simulink model "Kurs"  (R2024a)
settings: Solver=ode1  StartTime=0.0  StopTime=1.2  FixedStep=0.000001  RelTol=1e-3
InitFcn:
  | Kpr = 56;
  | Tpr = 0.002;
  | Rya = 1.78;
  | Tya = 0.16;
  | c = 0.56;
  | J = 0.05;
  | Kot = 0.054;
  | Koc = 0.09;
  | T1 = 0.0013;
  | T2 = 0.0165;
  | T4 = 0.207;
  | K1 = 6.74;
  | K2 = 3.12;
  | K3 = 0.874;
  | X1max = 3;
  | Y2max = 250;
  | Y4max = 90;
  | Z = 17;
  | treg = 0.001;
  | toy = 0.0001;
undefined symbols (not defined in the file or in its folder): Kaw, tre
libraries: slpidlib x5
(part 1 of 2)
settings Model: Creator=nicki  LastModifiedBy=nicki
settings RTWCC: GPUComputeCapability=3.5

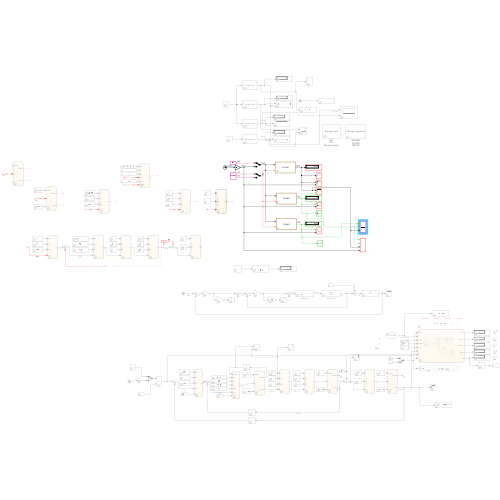
[thumbnail: Simulink's stored preview of the top-level diagram]
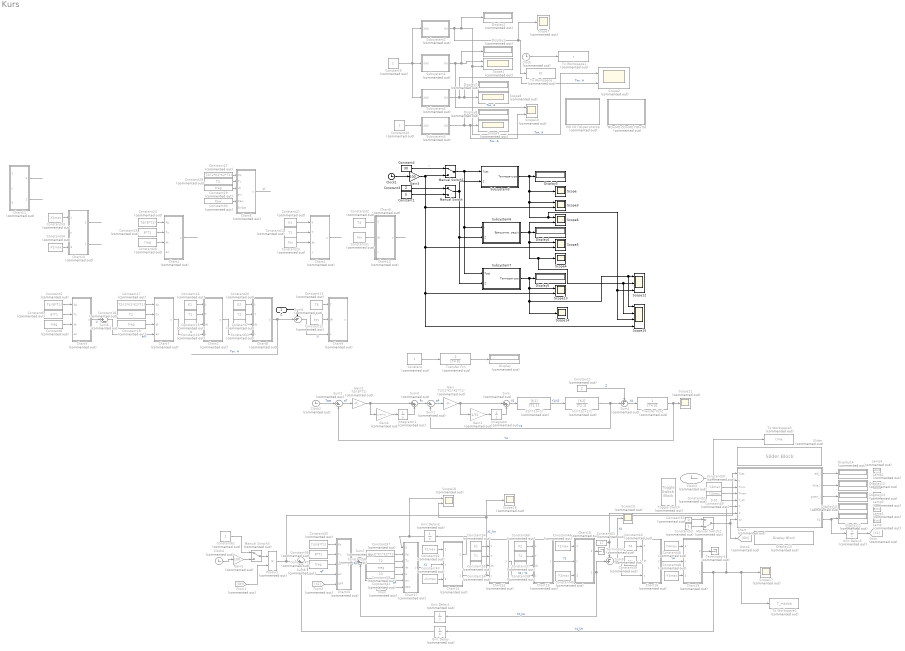
== system Kurs ==
  Z : Inport
  Chart : Stateflow chart  Commented=on  TreatAsAtomicUnit=on  SystemSampleTime=treg
      settings: PortSchema="{\"entries\":[{\"content\":{\"sides\":[{\"content\":{\"connectorIds\":[\"In8\",\"In1\",\"In2\",\"In3\",\"In5\",\"In4\",\"In6\",\"In7\"]},\"type\":\"ConnectorPlacement.EquallySpacedRectSide\",\"uuid\":\"2a18dcd6-4b0c-4a76-a20c-2dc316dd2b01\"},{\"content\":{\"connectorIds\":[\"Out1\",\"Out2\",\"Out3\",\"Out4\",\"Out5\"],\"side\":\"RIGHT\"},\"type\":\"ConnectorPlacement.EquallySpacedRectSide\",\"uuid\":\"9e7f62ff-8b1d-44fe-8b34-5f319205903d\"},{\"content\":{\"side\":\"TOP\"},\"type\":\"ConnectorPlacement.EquallySpacedRectSide\",\"uuid\":\"488e4df1-10a7-4056-869a-c48ac259fb0e\"}]},\"type\":\"ConnectorPlacement.EquallySpacedConnector\",\"uuid\":\"21634ba7-0beb-4d40-a7b7-ac3b35c407ea\"}],\"packageUris\":[\"http://schema.mathworks.com/mf0/Connector/R2020b\"],\"version\":\"1.0\"}"
  Chart1 : Stateflow chart  Commented=on  TreatAsAtomicUnit=on  SystemSampleTime=treg
  Chart10 : Stateflow chart  Commented=on  TreatAsAtomicUnit=on  SystemSampleTime=treg
      settings: PortSchema="{\"entries\":[{\"content\":{\"sides\":[{\"content\":{\"connectorIds\":[\"In1\",\"In2\",\"In3\"]},\"type\":\"ConnectorPlacement.EquallySpacedRectSide\",\"uuid\":\"06dc2d10-fdc8-420b-b9cd-f5fc9c52f6ec\"},{\"content\":{\"connectorIds\":[\"Out2\",\"Out1\"],\"side\":\"RIGHT\"},\"type\":\"ConnectorPlacement.EquallySpacedRectSide\",\"uuid\":\"6c618a25-ba21-4ff8-999c-a9529d925b85\"},{\"content\":{\"side\":\"TOP\"},\"type\":\"ConnectorPlacement.EquallySpacedRectSide\",\"uuid\":\"fb5392fe-c913-4872-919e-93e45aee3608\"}]},\"type\":\"ConnectorPlacement.EquallySpacedConnector\",\"uuid\":\"af73c6a6-6f26-4653-9043-b34907f5f2e4\"}],\"packageUris\":[\"http://schema.mathworks.com/mf0/Connector/R2020b\"],\"version\":\"1.0\"}"
  Chart11 : Stateflow chart  Commented=on  TreatAsAtomicUnit=on  SystemSampleTime=treg
      settings: PortSchema="{\"entries\":[{\"content\":{\"sides\":[{\"content\":{\"connectorIds\":[\"In1\",\"In2\",\"In3\"]},\"type\":\"ConnectorPlacement.EquallySpacedRectSide\",\"uuid\":\"06dc2d10-fdc8-420b-b9cd-f5fc9c52f6ec\"},{\"content\":{\"connectorIds\":[\"Out2\",\"Out1\"],\"side\":\"RIGHT\"},\"type\":\"ConnectorPlacement.EquallySpacedRectSide\",\"uuid\":\"6c618a25-ba21-4ff8-999c-a9529d925b85\"},{\"content\":{\"side\":\"TOP\"},\"type\":\"ConnectorPlacement.EquallySpacedRectSide\",\"uuid\":\"fb5392fe-c913-4872-919e-93e45aee3608\"}]},\"type\":\"ConnectorPlacement.EquallySpacedConnector\",\"uuid\":\"af73c6a6-6f26-4653-9043-b34907f5f2e4\"}],\"packageUris\":[\"http://schema.mathworks.com/mf0/Connector/R2020b\"],\"version\":\"1.0\"}"
  Chart12 : Stateflow chart  Commented=on  TreatAsAtomicUnit=on  SystemSampleTime=toy
  Chart13 : Stateflow chart  Commented=on  TreatAsAtomicUnit=on  SystemSampleTime=toy
  Chart14 : Stateflow chart  Commented=on  TreatAsAtomicUnit=on  SystemSampleTime=treg
      settings: PortSchema="{\"entries\":[{\"content\":{\"sides\":[{\"content\":{\"connectorIds\":[\"In1\",\"In2\",\"In3\"]},\"type\":\"ConnectorPlacement.EquallySpacedRectSide\",\"uuid\":\"06dc2d10-fdc8-420b-b9cd-f5fc9c52f6ec\"},{\"content\":{\"connectorIds\":[\"Out2\",\"Out1\"],\"side\":\"RIGHT\"},\"type\":\"ConnectorPlacement.EquallySpacedRectSide\",\"uuid\":\"6c618a25-ba21-4ff8-999c-a9529d925b85\"},{\"content\":{\"side\":\"TOP\"},\"type\":\"ConnectorPlacement.EquallySpacedRectSide\",\"uuid\":\"fb5392fe-c913-4872-919e-93e45aee3608\"}]},\"type\":\"ConnectorPlacement.EquallySpacedConnector\",\"uuid\":\"af73c6a6-6f26-4653-9043-b34907f5f2e4\"}],\"packageUris\":[\"http://schema.mathworks.com/mf0/Connector/R2020b\"],\"version\":\"1.0\"}"
  Chart15 : Stateflow chart  Commented=on  TreatAsAtomicUnit=on  SystemSampleTime=toy
  Chart16 : Stateflow chart  Commented=on  TreatAsAtomicUnit=on  SystemSampleTime=toy
  Chart17 : Stateflow chart  Commented=on  TreatAsAtomicUnit=on  SystemSampleTime=treg
      settings: PortSchema="{\"entries\":[{\"content\":{\"sides\":[{\"content\":{\"connectorIds\":[\"In5\",\"In1\",\"In2\",\"In3\",\"In6\",\"In4\",\"In7\"]},\"type\":\"ConnectorPlacement.EquallySpacedRectSide\",\"uuid\":\"b164ad06-1259-4e4e-9be1-6467b125c0e4\"},{\"content\":{\"connectorIds\":[\"Out1\"],\"side\":\"RIGHT\"},\"type\":\"ConnectorPlacement.EquallySpacedRectSide\",\"uuid\":\"0593e984-4c4d-48f3-925e-b61cefc7aa48\"},{\"content\":{\"side\":\"TOP\"},\"type\":\"ConnectorPlacement.EquallySpacedRectSide\",\"uuid\":\"e7a407e5-6ce2-46ef-876b-9c67a31d7a68\"}]},\"type\":\"ConnectorPlacement.EquallySpacedConnector\",\"uuid\":\"345a9212-fd2f-406e-95cd-4fdf60a3ef4b\"}],\"packageUris\":[\"http://schema.mathworks.com/mf0/Connector/R2020b\"],\"version\":\"1.0\"}"
  Chart18 : Stateflow chart  Commented=on  TreatAsAtomicUnit=on  SystemSampleTime=toy
      settings: PortSchema="{\"entries\":[{\"content\":{\"sides\":[{\"content\":{\"connectorIds\":[\"In1\",\"In2\",\"In3\"]},\"type\":\"ConnectorPlacement.EquallySpacedRectSide\",\"uuid\":\"06dc2d10-fdc8-420b-b9cd-f5fc9c52f6ec\"},{\"content\":{\"connectorIds\":[\"Out2\",\"Out1\"],\"side\":\"RIGHT\"},\"type\":\"ConnectorPlacement.EquallySpacedRectSide\",\"uuid\":\"6c618a25-ba21-4ff8-999c-a9529d925b85\"},{\"content\":{\"side\":\"TOP\"},\"type\":\"ConnectorPlacement.EquallySpacedRectSide\",\"uuid\":\"fb5392fe-c913-4872-919e-93e45aee3608\"}]},\"type\":\"ConnectorPlacement.EquallySpacedConnector\",\"uuid\":\"af73c6a6-6f26-4653-9043-b34907f5f2e4\"}],\"packageUris\":[\"http://schema.mathworks.com/mf0/Connector/R2020b\"],\"version\":\"1.0\"}"
  Chart19 : Stateflow chart  Commented=on  TreatAsAtomicUnit=on  SystemSampleTime=toy
      settings: PortSchema="{\"entries\":[{\"content\":{\"sides\":[{\"content\":{\"connectorIds\":[\"In1\",\"In2\",\"In3\"]},\"type\":\"ConnectorPlacement.EquallySpacedRectSide\",\"uuid\":\"06dc2d10-fdc8-420b-b9cd-f5fc9c52f6ec\"},{\"content\":{\"connectorIds\":[\"Out2\",\"Out1\"],\"side\":\"RIGHT\"},\"type\":\"ConnectorPlacement.EquallySpacedRectSide\",\"uuid\":\"6c618a25-ba21-4ff8-999c-a9529d925b85\"},{\"content\":{\"side\":\"TOP\"},\"type\":\"ConnectorPlacement.EquallySpacedRectSide\",\"uuid\":\"fb5392fe-c913-4872-919e-93e45aee3608\"}]},\"type\":\"ConnectorPlacement.EquallySpacedConnector\",\"uuid\":\"af73c6a6-6f26-4653-9043-b34907f5f2e4\"}],\"packageUris\":[\"http://schema.mathworks.com/mf0/Connector/R2020b\"],\"version\":\"1.0\"}"
  Chart2 : Stateflow chart  Commented=on  TreatAsAtomicUnit=on  SystemSampleTime=toy
  Chart20 : Stateflow chart  Commented=on  TreatAsAtomicUnit=on  SystemSampleTime=treg
  Chart3 : Stateflow chart  Commented=on  TreatAsAtomicUnit=on  SystemSampleTime=treg
  Chart4 : Stateflow chart  Commented=on  TreatAsAtomicUnit=on  SystemSampleTime=toy
  Chart5 : Stateflow chart  Commented=on  TreatAsAtomicUnit=on  SystemSampleTime=toy
  Chart6 : Stateflow chart  Commented=on  TreatAsAtomicUnit=on  SystemSampleTime=treg
      settings: PortSchema="{\"entries\":[{\"content\":{\"sides\":[{\"content\":{\"connectorIds\":[\"In1\",\"In2\",\"In3\",\"In4\",\"In6\",\"In5\"]},\"type\":\"ConnectorPlacement.EquallySpacedRectSide\",\"uuid\":\"b164ad06-1259-4e4e-9be1-6467b125c0e4\"},{\"content\":{\"connectorIds\":[\"Out1\"],\"side\":\"RIGHT\"},\"type\":\"ConnectorPlacement.EquallySpacedRectSide\",\"uuid\":\"0593e984-4c4d-48f3-925e-b61cefc7aa48\"},{\"content\":{\"side\":\"TOP\"},\"type\":\"ConnectorPlacement.EquallySpacedRectSide\",\"uuid\":\"e7a407e5-6ce2-46ef-876b-9c67a31d7a68\"}]},\"type\":\"ConnectorPlacement.EquallySpacedConnector\",\"uuid\":\"345a9212-fd2f-406e-95cd-4fdf60a3ef4b\"}],\"packageUris\":[\"http://schema.mathworks.com/mf0/Connector/R2020b\"],\"version\":\"1.0\"}"
  Chart7 : Stateflow chart  Commented=on  TreatAsAtomicUnit=on  SystemSampleTime=treg
  Chart8 : Stateflow chart  Commented=on  TreatAsAtomicUnit=on  SystemSampleTime=toy
  Chart9 : Stateflow chart  Commented=on  TreatAsAtomicUnit=on  SystemSampleTime=toy
  Clock{,2..4} (4 alike) : Clock  Commented=on
  Clock1 : Clock
  Constant{,9..10,52,61} (5 alike) : Constant  Commented=on
  Constant1 : Constant  Value=0
  Constant{11..12,16,23,31,38..39,56} (8 alike) : Constant  Commented=on  Value=toy
  Constant13 : Constant  Commented=on  Value=T4
  Constant14 : Constant  Commented=on  Value=K1
  Constant15 : Constant  Commented=on  Value=T1
  Constant17 : Constant  Commented=on  Value=T2/(2*K1*K2*T1)
  Constant{7,18,28,37,58} (5 alike) : Constant  Commented=on  Value=T2
  Constant{8,19,26,29,47,59} (6 alike) : Constant  Commented=on  Value=treg
  Constant2 : Constant  Commented=on  Value=Z
  Constant20 : Constant  Commented=on  Value=K2
  Constant21 : Constant  Commented=on  Value=K1
  Constant22 : Constant  Commented=on  Value=T1
  Constant24 : Constant  Commented=on  Value=T4/(8*T1)
  Constant25 : Constant  Commented=on  Value=8*T1
  Constant27 : Constant  Commented=on  Value=T2/(2*K1*K2*T1)
  Constant3 : Constant  Value=Z
  Constant30 : Constant  Commented=on  Value=Kaw
  Constant32 : Constant  Commented=on  Value=T4
  Constant33 : Constant  Commented=on  Value=X1max
  Constant34 : Constant  Commented=on  Value=-X1max
  Constant35 : Constant  Commented=on  Value=T4/(8*T1)
  Constant36 : Constant  Commented=on  Value=8*T1
  Constant4 : Constant  Value=30
  Constant40 : Constant  Commented=on  Value=T4
  Constant41 : Constant  Commented=on  Value=10
  Constant42 : Constant  Commented=on  Value=X1max
  Constant43 : Constant  Commented=on  Value=-X1max
  Constant44 : Constant  Commented=on  Value=Y2max
  Constant45 : Constant  Commented=on  Value=-Y2max
  Constant46 : Constant  Commented=on  Value=Y4max
  Constant48 : Constant  Commented=on  Value=-Y4max
  Constant49 : Constant  Commented=on  Value=Y4max
  Constant5 : Constant  Commented=on  Value=T4/(8*T1)
  Constant50 : Constant  Commented=on  Value=-Y4max
  Constant51 : Constant  Commented=on  Value=0.01
  Constant53 : Constant  Commented=on  Value=0
  Constant54 : Constant  Commented=on  Value=K1
  Constant55 : Constant  Commented=on  Value=T1
  Constant57 : Constant  Commented=on  Value=T2/(2*K1*K2*T1)
  Constant6 : Constant  Commented=on  Value=8*T1
  Constant60 : Constant  Commented=on  Value=K2
  Constant62 : Constant  Commented=on  Value=17
  Display{,1..2,7..8,10..14} (10 alike) : Display  Commented=on
  Display15 : DisplayBlock  Commented=on  LabelPosition=Hide  Transparency=1
  Display3 : Display
  Display4 : Display
  Display5 : Display
  From : From  Commented=on  GotoTag=X1
  From1 : From  Commented=on  GotoTag=ON
  From2 : From  Commented=on  GotoTag=X1
  Gain : Gain  Commented=on  Gain=T2/(2*K1*K2*T1)
  Gain1 : Gain  Commented=on  Gain=1/T2
  Gain2 : Gain  Commented=on  Gain=T4/(8*T1)
  Gain3 : Gain  Gain=100
  Gain4 : Gain  Commented=on  Gain=1/(8*T1)
  Gain5 : Gain  Commented=on  Gain=100
  Goto : Goto  Commented=on  GotoTag=X1
  Goto1 : Goto  Commented=on  GotoTag=ON
  Integrator : Integrator  Commented=on
  Integrator1 : Integrator  Commented=on
  Lamp : LampBlock  Commented=on  LabelPosition=Hide  Icon=Check1
  Lamp1 : LampBlock  Commented=on  LabelPosition=Hide  Icon=Check1
  Lamp2 : LampBlock  Commented=on  LabelPosition=Hide
  Lamp3 : LampBlock  Commented=on  LabelPosition=Hide
  Lamp4 : LampBlock  Commented=on  LabelPosition=Hide
  Manual Switch : ManualSwitch
  Manual Switch1 : ManualSwitch
  Manual Switch2 : ManualSwitch  Commented=on  CurrentSetting=0
  Manual Switch3 : ManualSwitch  Commented=on
  Product : Product  Commented=on
  Scope : Scope
  Scope{1..2,10,18} (4 alike) : Scope  Commented=on  NumInputPorts=2
  Scope{7..9,11,16..17,19} (7 alike) : Scope  Commented=on
  Scope12 : Scope  NumInputPorts=3
  Scope{3,5..6,13} (4 alike) : Scope  NumInputPorts=2
  Scope14 : Scope
  Scope15 : Scope  NumInputPorts=4
  Scope4 : Scope
  Slider : SliderBlock  Commented=on  ScaleMin=-100
  Subsystem1 : Subsystem  Commented=on  mask{Kpr=Kpr, Tpr=Tpr, Rya=Rya, Tya=Tya, Cm=c, Ce=c, Kot=Kot, Koc=Koc, treg=1/1000, toy=1 / 10000}
      mask prompts: Kpr "Коэффициент усиления преобразователя"; Tpr "Постоянная времени преобразователя"; Rya "Коэффициент усиления тока (1/Rya)"; Tya "Постоянная времени тока"; Cm "Постоянный конструктивный коэффициент (коэффициент связи)"; Ce "Постоянный конструктивный коэффициент (u = Ce*w)"; Kot "Коэффициент обратной связи тока"; Koc "Коэффициент обратной связи угловой скорости"; treg "Шаг дискретизации регуляторов"; toy "Шаг дискретизации ОУ"
      mask Display: disp('Контур тока');
  Subsystem2 : Subsystem  Commented=on  mask{Kpr=Kpr, Tpr=Tpr, Rya=Rya, Tya=Tya, Cm=c, Ce=c, Kot=Kot, Koc=Koc, treg=1/1000, toy=1 / 10000}
      mask prompts: Kpr "Коэффициент усиления преобразователя"; Tpr "Постоянная времени преобразователя"; Rya "Коэффициент усиления тока (1/Rya)"; Tya "Постоянная времени тока"; Cm "Постоянный конструктивный коэффициент (коэффициент связи)"; Ce "Постоянный конструктивный коэффициент (u = Ce*w)"; Kot "Коэффициент обратной связи тока"; Koc "Коэффициент обратной связи угловой скорости"; treg "Шаг дискретизации регуляторов"; toy "Шаг дискретизации ОУ"
      mask Display: disp('Контур тока');
  Subsystem3 : Subsystem
      mask Display: disp('СО+МО');
  Subsystem4 : Subsystem  Commented=on  mask{Kpr=Kpr, Tpr=Tpr, Rya=Rya, Tya=Tya, Cm=c, Ce=c, Kot=Kot, Koc=Koc, treg=1/1000, toy=1 / 10000}
      mask prompts: Kpr "Коэффициент усиления преобразователя"; Tpr "Постоянная времени преобразователя"; Rya "Коэффициент усиления тока (1/Rya)"; Tya "Постоянная времени тока"; Cm "Постоянный конструктивный коэффициент (коэффициент связи)"; Ce "Постоянный конструктивный коэффициент (u = Ce*w)"; Kot "Коэффициент обратной связи тока"; Koc "Коэффициент обратной связи угловой скорости"; treg "Шаг дискретизации регуляторов"; toy "Шаг дискретизации ОУ"
      mask Display: disp('Контур тока');
  Subsystem5 : Subsystem  Commented=on  mask{Kpr=Kpr, Tpr=Tpr, Rya=Rya, Tya=Tya, Cm=c, Ce=c, Kot=Kot, Koc=Koc, treg=1/1000, toy=1 / 10000}
      mask prompts: Kpr "Коэффициент усиления преобразователя"; Tpr "Постоянная времени преобразователя"; Rya "Коэффициент усиления тока (1/Rya)"; Tya "Постоянная времени тока"; Cm "Постоянный конструктивный коэффициент (коэффициент связи)"; Ce "Постоянный конструктивный коэффициент (u = Ce*w)"; Kot "Коэффициент обратной связи тока"; Koc "Коэффициент обратной связи угловой скорости"; treg "Шаг дискретизации регуляторов"; toy "Шаг дискретизации ОУ"
      mask Display: disp('ПИ (дискрет)');
  Subsystem6 : Subsystem
      mask Display: disp('СО+МО');
  Subsystem7 : Subsystem
      mask Display: disp('СО+МО');
  Sum : Sum  Commented=on  Inputs=|++
  Sum{1..2,5,7..8} (5 alike) : Sum  Commented=on  Inputs=|+-
  Sum3 : Sum  Commented=on  Inputs=|++
  Sum4 : Sum  Commented=on  Inputs=-+|
  Sum6 : Sum  Commented=on  Inputs=-+|
  Sum9 : Sum  Commented=on  Inputs=-+|
  Terminator : Terminator  Commented=on
  Terminator1 : Terminator  Commented=on
  To Workspace : ToWorkspace  Commented=on  VariableName=Kt  SampleTime=0.001
  To Workspace1 : ToWorkspace  Commented=on  VariableName=t  SampleTime=0.001
  To Workspace2 : ToWorkspace  Commented=on  VariableName=T_matlab  SampleTime=0.002
  To Workspace3 : ToWorkspace  Commented=on  VariableName=time  SampleTime=0.002
  Toggle Switch : ToggleSwitchBlock  Commented=on
      settings: Values={{'Off', 'On'}, [17 0]}
  Transfer Fcn : TransferFcn  Commented=on  Denominator=[T4 0]
  Transfer Fcn1 : TransferFcn  Commented=on  Denominator=[T4 0]
  Unit Delay{,1..3} (4 alike) : UnitDelay  Commented=on  SampleTime=treg  HasFrameUpgradeWarning=on
  k1/(T1s+1) : TransferFcn  Commented=on  Numerator=[K1]  Denominator=[T1 1]
  k1/(T1s+1)1 : TransferFcn  Commented=on  Numerator=[K2]  Denominator=[T2 1]
  МО СО ПИ-регулятор : Subsystem  Commented=on
      mask Display: disp('Контур тока');
  МО+МО СО+МО ПИ+ПИ : Subsystem  Commented=on
      mask Display: disp('Контур скорости');
  wires:
  Subsystem4/1(I(t)) -> Scope2/2, Display7/1, Scope8/1  "Ток, А"
  Subsystem5/1(I(t)) -> Display8/1, Scope10/2, Scope9/1  "Ток, А"
  Constant10/1 -> Subsystem5/1(i0(t))
  Subsystem1/1(I(t)) -> Scope10/1, Display1/1, Scope1/1  "Ток, А"
  Constant9/1 -> Subsystem4/1(i0(t)), Subsystem2/1(i0(t)), Subsystem1/1(i0(t))
  Subsystem2/1(I(t)) -> Scope7/1, To Workspace/1, Display2/1, Scope1/2, Scope2/1  "Ток, А"
  Clock/1 -> To Workspace1/1
  Manual Switch1/1 -> Subsystem7/1(Tset), Subsystem6/1(i), Subsystem3/1(Tset)
  Manual Switch/1 -> Subsystem7/2(Z), Subsystem6/2(Z), Subsystem3/2(Z)
  Constant1/1 -> Manual Switch/2
  Constant3/1 -> Manual Switch/1
  Subsystem3/1(Температура) -> Display3/1, Scope15/3, Scope12/3, Scope6/1, Scope3/1, Scope/1
  Constant4/1 -> Manual Switch1/1  "i"
  Subsystem6/1("Вращение, рад/с") -> Scope6/2, Scope15/2, Scope12/2, Scope4/1, Scope5/1, Display4/1
  Constant/1 -> Transfer Fcn/1
  Transfer Fcn/1 -> Display/1
  Integrator1/1 -> Sum3/2
  Gain2/1 -> Sum3/1, Gain4/1
  Gain4/1 -> Integrator1/1
  k1/(T1s+1)/1 -> k1/(T1s+1)1/1  "Y1/X2"
  Gain/1 -> Gain1/1, Sum/1
  Constant2/1 -> Sum4/1  "Z"
  Sum4/1 -> Transfer Fcn1/1  "X4"
  Transfer Fcn1/1 -> Scope11/1, Sum2/2  "Y4"
  Sum1/1 -> Gain/1  "eP"
  Clock2/1 -> Sum2/1  "Tset"
  Sum2/1 -> Gain2/1  "eT"
  Gain1/1 -> Integrator/1
  Sum/1 -> k1/(T1s+1)/1  "X1"
  k1/(T1s+1)1/1 -> Sum4/2, Sum1/2  "Y2"
  Integrator/1 -> Sum/2
  Sum3/1 -> Sum1/1  "Pn"
  Subsystem7/1(Температура) -> Scope14/1, Scope15/1, Scope12/1, Scope13/1, Display5/1
  Clock1/1 -> Gain3/1
  Chart7/1(y) -> Chart2/4(x)  "U"
  Chart2/1(y) -> Chart8/4(x)
  ? -> Sum5/2
  Chart8/1(y) -> Sum6/2  "Ток, А"
  ? -> Chart3/4(err)  "e(i)"
  Constant18/1 -> Chart7/2(Tu)
  Constant12/1 -> Chart9/2(dt)
  Constant11/1 -> Chart8/3(dt)
  Constant20/1 -> Chart8/1(k)
  Constant13/1 -> Chart9/1(T)
  Constant19/1 -> Chart7/3(dt)
  Constant15/1 -> Chart2/2(T)
  Constant16/1 -> Chart2/3(dt)
  Z/1 -> Sum6/1
  Constant7/1 -> Chart8/2(T)
  Constant8/1 -> Chart3/3(dt)
  Constant5/1 -> Chart3/1(Kp)
  Sum6/1 -> Chart9/3(x)  "U"
  Constant17/1 -> Chart7/1(Kp)
  Chart3/1(y) -> Sum5/1  "U"
  Sum5/1 -> Chart7/4(err)  "e(i)"
  Constant6/1 -> Chart3/2(Tu)
  Constant14/1 -> Chart2/1(k)
  Constant21/1 -> Chart4/1(k)
  Constant22/1 -> Chart4/2(T)
  Constant23/1 -> Chart4/3(dt)
  ? -> Chart4/4(x)
  Chart4/1(y) -> ?
  Constant24/1 -> Chart1/1(Kp)
  Constant25/1 -> Chart1/2(Tu)
  Constant26/1 -> Chart1/3(dt)
  ? -> Chart1/4(err)
  Chart1/1(y) -> ?
  Constant27/1 -> Chart6/1(Kp)
  Constant28/1 -> Chart6/2(Tu)
  Constant29/1 -> Chart6/3(dt)
  Constant30/1 -> Chart6/6(Kaw)
  ? -> Chart6/4(err)
  ? -> Chart6/5(ErrSat)
  Chart6/1(y) -> ?  "U"
  Constant32/1 -> Chart5/1(T)
  Constant31/1 -> Chart5/2(dt)
  Chart5/1(y) -> ?
  ? -> Chart5/3(x)
  Constant34/1 -> Chart10/3(Ymin)
  Constant33/1 -> Chart10/1(Ymax)
  ? -> Chart10/2(y)  "U"
  Chart10/2(ErrSat) -> ?
  Chart10/1(y_lim) -> ?
  Chart11/1(y_lim) -> ?
  ? -> Chart11/2(y)  "U"
  Chart11/2(ErrSat) -> ?
  Gain3/1 -> Manual Switch1/2, Scope3/2, Scope15/4, Scope13/2, Scope5/2
  Constant50/1 -> Chart/2(Tmin)
  Product/1 -> Chart/8(Tset), Sum8/1
  Constant52/1 -> Manual Switch2/2
  From2/1 -> Chart20/5(OFF)
  From1/1 -> Product/2
  Chart/1(red_l) -> Display14/1
  Clock3/1 -> To Workspace3/1, Chart/1(t)
  Constant51/1 -> Chart/5(T_dz)
  Unit Delay3/1 -> Goto/1
  Chart14/2(ErrSat) -> Unit Delay2/1
  Constant48/1 -> Chart19/3(Ymin)
  Constant49/1 -> Chart/3(Tmax)
  Constant53/1 -> Manual Switch2/1
  Chart19/2(ErrSat) -> Terminator1/1
  Chart/3(green_l) -> Display13/1
  Unit Delay1/1 -> Sum7/2
  Chart18/2(ErrSat) -> Terminator/1
  Clock4/1 -> Gain5/1
  Constant37/1 -> Chart15/2(T)
  Constant44/1 -> Chart18/1(Ymax)
  Constant43/1 -> Chart14/3(Ymin)
  From/1 -> Chart17/7(OFF)
  Sum8/1 -> Chart20/4(err)  "eT"
  Constant54/1 -> Chart12/1(k)
  Constant46/1 -> Chart19/1(Ymax)
  Chart19/1(y_lim) -> To Workspace2/1, Scope17/1, Chart/4(T), Unit Delay/1  "Y4_lim"
  Chart16/1(y) -> Chart19/2(y)  "Y4"
  Constant55/1 -> Chart12/2(T)
  Manual Switch2/1 -> Goto1/1, Chart/7(on)
  Constant60/1 -> Chart15/1(k)
  Chart15/1(y) -> Chart18/2(y)  "Y2"
  Constant57/1 -> Chart17/1(Kp)
  Constant56/1 -> Chart12/3(dt)
  Constant40/1 -> Chart16/1(T)
  Unit Delay2/1 -> Scope18/1, Chart17/5(ErrSat)
  Constant59/1 -> Chart17/3(dt)
  Constant58/1 -> Chart17/2(Tu)
  Chart/4(error) -> Display10/1
  Constant42/1 -> Chart14/1(Ymax)
  Chart/5(X1) -> Display11/1, Unit Delay3/1
  Unit Delay/1 -> Sum8/2
  Constant45/1 -> Chart18/3(Ymin)
  Chart14/1(y_lim) -> Scope18/2, Scope16/1, Chart12/4(x)  "X1_lim"
  Chart18/1(y_lim) -> Unit Delay1/1, Sum9/2  "Y2_lim"
  Constant39/1 -> Chart16/2(dt)
  Chart17/1(y) -> Chart14/2(y)  "X1"
  Constant38/1 -> Chart15/3(dt)
  Constant47/1 -> Chart20/3(dt)
  Constant62/1 -> Sum9/1, Chart/6(Z)
  Chart12/1(y) -> Chart15/4(x)  "X2 / Y1"
  Constant36/1 -> Chart20/2(Tu)
  Constant35/1 -> Chart20/1(Kp)
  Chart20/1(y) -> Sum7/1  "Pn"
  Constant41/1 -> Chart17/6(Kaw)
  Sum9/1 -> Scope19/1, Chart16/3(x)  "X4"
  Sum7/1 -> Chart17/4(err)  "eP"
  Chart/2(blue_l) -> Display12/1
  Manual Switch3/1 -> Product/1
  Gain5/1 -> Manual Switch3/2
  Constant61/1 -> Manual Switch3/1

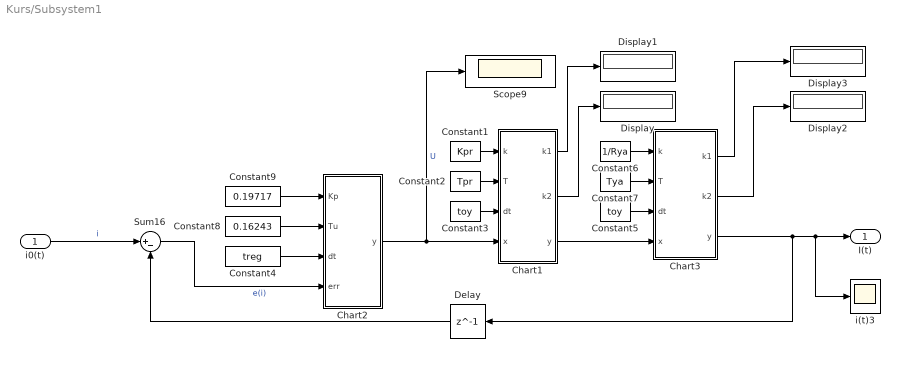
== system Kurs/Subsystem1 ==
  i0(t) : Inport
  Chart1 : Stateflow chart  TreatAsAtomicUnit=on  SystemSampleTime=toy
      settings: PortSchema="{\"entries\":[{\"content\":{\"sides\":[{\"content\":{\"connectorIds\":[\"In1\",\"In2\",\"In3\",\"In4\"]},\"type\":\"ConnectorPlacement.EquallySpacedRectSide\",\"uuid\":\"36dbee36-691d-4a1c-ac9a-2338e443d86d\"},{\"content\":{\"connectorIds\":[\"Out2\",\"Out3\",\"Out1\"],\"side\":\"RIGHT\"},\"type\":\"ConnectorPlacement.EquallySpacedRectSide\",\"uuid\":\"ede5d785-9ed8-4f22-af08-79b1e7897644\"},{\"content\":{\"side\":\"TOP\"},\"type\":\"ConnectorPlacement.EquallySpacedRectSide\",\"uuid\":\"89777bdd-54fe-413f-92dc-46747ee34626\"}]},\"type\":\"ConnectorPlacement.EquallySpacedConnector\",\"uuid\":\"a256a943-0a0c-4b11-963e-36f9b93f9ce8\"}],\"packageUris\":[\"http://schema.mathworks.com/mf0/Connector/R2020b\"],\"version\":\"1.0\"}"
  Chart2 : Stateflow chart  TreatAsAtomicUnit=on  SystemSampleTime=treg
  Chart3 : Stateflow chart  TreatAsAtomicUnit=on  SystemSampleTime=toy
      settings: PortSchema="{\"entries\":[{\"content\":{\"sides\":[{\"content\":{\"connectorIds\":[\"In1\",\"In2\",\"In3\",\"In4\"]},\"type\":\"ConnectorPlacement.EquallySpacedRectSide\",\"uuid\":\"36dbee36-691d-4a1c-ac9a-2338e443d86d\"},{\"content\":{\"connectorIds\":[\"Out2\",\"Out3\",\"Out1\"],\"side\":\"RIGHT\"},\"type\":\"ConnectorPlacement.EquallySpacedRectSide\",\"uuid\":\"ede5d785-9ed8-4f22-af08-79b1e7897644\"},{\"content\":{\"side\":\"TOP\"},\"type\":\"ConnectorPlacement.EquallySpacedRectSide\",\"uuid\":\"89777bdd-54fe-413f-92dc-46747ee34626\"}]},\"type\":\"ConnectorPlacement.EquallySpacedConnector\",\"uuid\":\"a256a943-0a0c-4b11-963e-36f9b93f9ce8\"}],\"packageUris\":[\"http://schema.mathworks.com/mf0/Connector/R2020b\"],\"version\":\"1.0\"}"
  Constant1 : Constant  Value=Kpr
  Constant2 : Constant  Value=Tpr
  Constant3 : Constant  Value=toy
  Constant4 : Constant  Value=treg
  Constant5 : Constant  Value=toy
  Constant6 : Constant  Value=1/Rya
  Constant7 : Constant  Value=Tya
  Constant8 : Constant  Value=0.16243
  Constant9 : Constant  Value=0.19717
  Delay : Delay  DelayLength=1  SampleTime=toy
  Display{,1..3} (4 alike) : Display
  Scope9 : Scope
  Sum16 : Sum  Inputs=|+-
  i(t)3 : Scope
  I(t) : Outport
  wires:
  Sum16/1 -> Chart2/4(err)  "e(i)"
  Chart2/1(y) -> Chart1/4(x), Scope9/1  "U"
  i0(t)/1 -> Sum16/1  "i"
  Chart3/1(y) -> Delay/1, i(t)3/1, I(t)/1
  Constant7/1 -> Chart3/2(T)
  Constant6/1 -> Chart3/1(k)
  Constant5/1 -> Chart3/3(dt)
  Chart1/1(y) -> Chart3/4(x)
  Constant1/1 -> Chart1/1(k)
  Constant2/1 -> Chart1/2(T)
  Constant3/1 -> Chart1/3(dt)
  Delay/1 -> Sum16/2
  Chart1/3(k2) -> Display/1
  Chart1/2(k1) -> Display1/1
  Chart3/3(k2) -> Display2/1
  Chart3/2(k1) -> Display3/1
  Constant4/1 -> Chart2/3(dt)
  Constant8/1 -> Chart2/2(Tu)
  Constant9/1 -> Chart2/1(Kp)

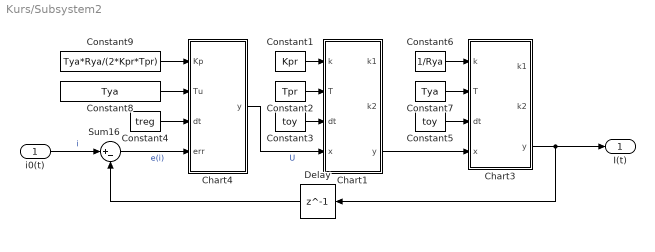
== system Kurs/Subsystem2 ==
  i0(t) : Inport
  Chart1 : Stateflow chart  TreatAsAtomicUnit=on  SystemSampleTime=toy
      settings: PortSchema="{\"entries\":[{\"content\":{\"sides\":[{\"content\":{\"connectorIds\":[\"In1\",\"In2\",\"In3\",\"In4\"]},\"type\":\"ConnectorPlacement.EquallySpacedRectSide\",\"uuid\":\"36dbee36-691d-4a1c-ac9a-2338e443d86d\"},{\"content\":{\"connectorIds\":[\"Out2\",\"Out3\",\"Out1\"],\"side\":\"RIGHT\"},\"type\":\"ConnectorPlacement.EquallySpacedRectSide\",\"uuid\":\"ede5d785-9ed8-4f22-af08-79b1e7897644\"},{\"content\":{\"side\":\"TOP\"},\"type\":\"ConnectorPlacement.EquallySpacedRectSide\",\"uuid\":\"89777bdd-54fe-413f-92dc-46747ee34626\"}]},\"type\":\"ConnectorPlacement.EquallySpacedConnector\",\"uuid\":\"a256a943-0a0c-4b11-963e-36f9b93f9ce8\"}],\"packageUris\":[\"http://schema.mathworks.com/mf0/Connector/R2020b\"],\"version\":\"1.0\"}"
  Chart3 : Stateflow chart  TreatAsAtomicUnit=on  SystemSampleTime=toy
      settings: PortSchema="{\"entries\":[{\"content\":{\"sides\":[{\"content\":{\"connectorIds\":[\"In1\",\"In2\",\"In3\",\"In4\"]},\"type\":\"ConnectorPlacement.EquallySpacedRectSide\",\"uuid\":\"36dbee36-691d-4a1c-ac9a-2338e443d86d\"},{\"content\":{\"connectorIds\":[\"Out2\",\"Out3\",\"Out1\"],\"side\":\"RIGHT\"},\"type\":\"ConnectorPlacement.EquallySpacedRectSide\",\"uuid\":\"ede5d785-9ed8-4f22-af08-79b1e7897644\"},{\"content\":{\"side\":\"TOP\"},\"type\":\"ConnectorPlacement.EquallySpacedRectSide\",\"uuid\":\"89777bdd-54fe-413f-92dc-46747ee34626\"}]},\"type\":\"ConnectorPlacement.EquallySpacedConnector\",\"uuid\":\"a256a943-0a0c-4b11-963e-36f9b93f9ce8\"}],\"packageUris\":[\"http://schema.mathworks.com/mf0/Connector/R2020b\"],\"version\":\"1.0\"}"
  Chart4 : Stateflow chart  TreatAsAtomicUnit=on  SystemSampleTime=treg
  Constant1 : Constant  Value=Kpr
  Constant2 : Constant  Value=Tpr
  Constant3 : Constant  Value=toy
  Constant4 : Constant  Value=treg
  Constant5 : Constant  Value=toy
  Constant6 : Constant  Value=1/Rya
  Constant7 : Constant  Value=Tya
  Constant8 : Constant  Value=Tya
  Constant9 : Constant  Value=Tya*Rya/(2*Kpr*Tpr)
  Delay : Delay  DelayLength=1  SampleTime=toy
  Sum16 : Sum  Inputs=|+-
  I(t) : Outport
  wires:
  Sum16/1 -> Chart4/4(err)  "e(i)"
  Chart4/1(y) -> Chart1/4(x)  "U"
  i0(t)/1 -> Sum16/1  "i"
  Chart3/1(y) -> I(t)/1, Delay/1
  Constant7/1 -> Chart3/2(T)
  Constant6/1 -> Chart3/1(k)
  Constant5/1 -> Chart3/3(dt)
  Chart1/1(y) -> Chart3/4(x)
  Constant1/1 -> Chart1/1(k)
  Constant2/1 -> Chart1/2(T)
  Constant3/1 -> Chart1/3(dt)
  Delay/1 -> Sum16/2
  Constant4/1 -> Chart4/3(dt)
  Constant8/1 -> Chart4/2(Tu)
  Constant9/1 -> Chart4/1(Kp)

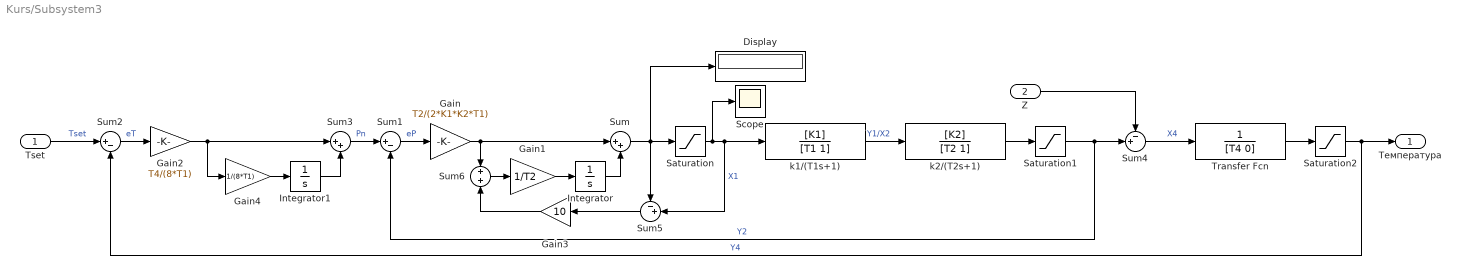
== system Kurs/Subsystem3 ==
  Tset : Inport
  Z : Inport  Port=2
  Display : Display
  Gain : Gain  Gain=T2/(2*K1*K2*T1)
  Gain1 : Gain  Gain=1/T2
  Gain2 : Gain  Gain=T4/(8*T1)
  Gain3 : Gain  Gain=10
  Gain4 : Gain  Gain=1/(8*T1)
  Integrator : Integrator
  Integrator1 : Integrator
  Saturation : Saturate  UpperLimit=X1max  LowerLimit=-X1max
  Saturation1 : Saturate  UpperLimit=Y2max  LowerLimit=-Y2max
  Saturation2 : Saturate  UpperLimit=Y4max  LowerLimit=-Y4max
  Scope : Scope
  Sum : Sum  Inputs=|++
  Sum1 : Sum  Inputs=|+-
  Sum2 : Sum  Inputs=|+-
  Sum3 : Sum  Inputs=|++
  Sum4 : Sum  Inputs=-+|
  Sum5 : Sum  Inputs=-+|
  Sum6 : Sum
  Transfer Fcn : TransferFcn  Denominator=[T4 0]
  k1/(T1s+1) : TransferFcn  Numerator=[K1]  Denominator=[T1 1]
  k2/(T2s+1) : TransferFcn  Numerator=[K2]  Denominator=[T2 1]
  Температура : Outport
  wires:
  Gain1/1 -> Integrator/1
  Gain/1 -> Sum6/1, Sum/1
  Integrator/1 -> Sum/2
  k2/(T2s+1)/1 -> Saturation1/1
  Sum/1 -> Display/1, Saturation/1, Sum5/1
  Sum1/1 -> Gain/1  "eP"
  Sum2/1 -> Gain2/1  "eT"
  Tset/1 -> Sum2/1  "Tset"
  Sum3/1 -> Sum1/1  "Pn"
  Integrator1/1 -> Sum3/2
  Gain4/1 -> Integrator1/1
  Gain2/1 -> Sum3/1, Gain4/1
  k1/(T1s+1)/1 -> k2/(T2s+1)/1  "Y1/X2"
  Sum4/1 -> Transfer Fcn/1  "X4"
  Z/1 -> Sum4/1
  Saturation/1 -> Scope/1, k1/(T1s+1)/1, Sum5/2  "X1"
  Sum6/1 -> Gain1/1
  Sum5/1 -> Gain3/1
  Gain3/1 -> Sum6/2
  Transfer Fcn/1 -> Saturation2/1
  Saturation1/1 -> Sum4/2, Sum1/2  "Y2"
  Saturation2/1 -> Температура/1, Sum2/2  "Y4"

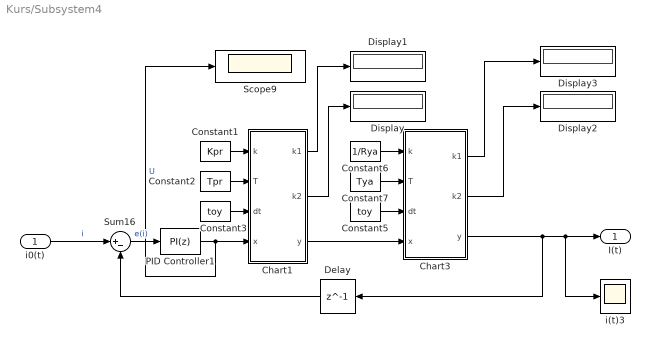
== system Kurs/Subsystem4 ==
  i0(t) : Inport
  Chart1 : Stateflow chart  TreatAsAtomicUnit=on  SystemSampleTime=toy
      settings: PortSchema="{\"entries\":[{\"content\":{\"sides\":[{\"content\":{\"connectorIds\":[\"In1\",\"In2\",\"In3\",\"In4\"]},\"type\":\"ConnectorPlacement.EquallySpacedRectSide\",\"uuid\":\"36dbee36-691d-4a1c-ac9a-2338e443d86d\"},{\"content\":{\"connectorIds\":[\"Out2\",\"Out3\",\"Out1\"],\"side\":\"RIGHT\"},\"type\":\"ConnectorPlacement.EquallySpacedRectSide\",\"uuid\":\"ede5d785-9ed8-4f22-af08-79b1e7897644\"},{\"content\":{\"side\":\"TOP\"},\"type\":\"ConnectorPlacement.EquallySpacedRectSide\",\"uuid\":\"89777bdd-54fe-413f-92dc-46747ee34626\"}]},\"type\":\"ConnectorPlacement.EquallySpacedConnector\",\"uuid\":\"a256a943-0a0c-4b11-963e-36f9b93f9ce8\"}],\"packageUris\":[\"http://schema.mathworks.com/mf0/Connector/R2020b\"],\"version\":\"1.0\"}"
  Chart3 : Stateflow chart  TreatAsAtomicUnit=on  SystemSampleTime=toy
      settings: PortSchema="{\"entries\":[{\"content\":{\"sides\":[{\"content\":{\"connectorIds\":[\"In1\",\"In2\",\"In3\",\"In4\"]},\"type\":\"ConnectorPlacement.EquallySpacedRectSide\",\"uuid\":\"36dbee36-691d-4a1c-ac9a-2338e443d86d\"},{\"content\":{\"connectorIds\":[\"Out2\",\"Out3\",\"Out1\"],\"side\":\"RIGHT\"},\"type\":\"ConnectorPlacement.EquallySpacedRectSide\",\"uuid\":\"ede5d785-9ed8-4f22-af08-79b1e7897644\"},{\"content\":{\"side\":\"TOP\"},\"type\":\"ConnectorPlacement.EquallySpacedRectSide\",\"uuid\":\"89777bdd-54fe-413f-92dc-46747ee34626\"}]},\"type\":\"ConnectorPlacement.EquallySpacedConnector\",\"uuid\":\"a256a943-0a0c-4b11-963e-36f9b93f9ce8\"}],\"packageUris\":[\"http://schema.mathworks.com/mf0/Connector/R2020b\"],\"version\":\"1.0\"}"
  Constant1 : Constant  Value=Kpr
  Constant2 : Constant  Value=Tpr
  Constant3 : Constant  Value=toy
  Constant5 : Constant  Value=toy
  Constant6 : Constant  Value=1/Rya
  Constant7 : Constant  Value=Tya
  Delay : Delay  DelayLength=1  SampleTime=toy
  Display{,1..3} (4 alike) : Display
  PID Controller1 : slpidlib/PID Controller  Controller=PI  Form=Parallel  TimeDomain=Discrete-time  UseExternalTs=off  SampleTime=treg  IntegratorMethod=Forward Euler  FilterMethod=Forward Euler  ControllerParametersSource=internal  P=Tya*Rya/(2*Kpr*Tpr)  I=1/Tya  UseKiTs=off  D=-544.981619005016  UseExternalDerivativeSource=off  N=0.000737427491300299  UseFilter=on  TunerSelectOption=Transfer Function Based (PID Tuner App)  InitialConditionSource=internal  InitialConditionForIntegrator=0  InitialConditionForFilter=0  DifferentiatorICPrevScaledInput=0  ExternalReset=none  TrackingMode=off  Kt=1  LimitOutput=off  SatLimitsSource=internal  UpperSaturationLimit=12  LowerSaturationLimit=-12  LinearizeAsGain=on  AntiWindupMode=none  Kb=1  LimitIntegrator=off  UpperIntegratorSaturationLimit=inf  LowerIntegratorSaturationLimit=-inf  POutMin=[]  POutMax=[]  IOutMin=[]  IOutMax=[]  DOutMin=[]  DOutMax=[]  NOutMin=[]  NOutMax=[]  SumOutMin=[]  SumOutMax=[]  SaturationOutMin=[]  SaturationOutMax=[]  PParamMin=[]  PParamMax=[]  IParamMin=[]  IParamMax=[]  DParamMin=[]  DParamMax=[]  NParamMin=[]  NParamMax=[]  KbParamMin=[]  KbParamMax=[]  KtParamMin=[]  KtParamMax=[]  KbOutMin=[]  KbOutMax=[]  KtOutMin=[]  KtOutMax=[]  IntegratorOutMin=[]  IntegratorOutMax=[]  FilterOutMin=[]  FilterOutMax=[]  SumI1OutMin=[]  SumI1OutMax=[]  SumI2OutMin=[]  SumI2OutMax=[]  SumI3OutMin=[]  SumI3OutMax=[]  SumI4OutMin=[]  SumI4OutMax=[]  SumDOutMin=[]  SumDOutMax=[]  DifferentiatorOutMin=[]  DifferentiatorOutMax=[]  FilterDiffOutCoefMin=[]  FilterDiffOutCoefMax=[]  ReciprocalOutMin=[]  ReciprocalOutMax=[]  SumDenOutMin=[]  SumDenOutMax=[]  SumNumOutMin=[]  SumNumOutMax=[]  DivideOutMin=[]  DivideOutMax=[]  UdiffTsProdOutMin=[]  UdiffTsProdOutMax=[]  NTsProdOutMin=[]  NTsProdOutMax=[]  UintegralTsProdOutMin=[]  UintegralTsProdOutMax=[]  UngainTsProdOutMin=[]  UngainTsProdOutMax=[]  ClampingZeroOutDataTypeStr=Inherit: Inherit via back propagation  ClampingZeroOutMin=[]  ClampingZeroOutMax=[]  FilterDenConstantOutDataTypeStr=Inherit: Inherit via back propagation  FilterDenConstantOutMin=[]  FilterDenConstantOutMax=[]  PCopyOutDataTypeStr=Inherit: Inherit via back propagation  PCopyOutMin=[]  PCopyOutMax=[]  NCopyOutDataTypeStr=Inherit: Inherit via back propagation  NCopyOutMin=[]  NCopyOutMax=[]  IntegratorContinuousStateAttributes=''  IntegratorStateMustResolveToSignalObject=off  IntegratorRTWStateStorageClass=Auto  FilterContinuousStateAttributes=''  FilterStateMustResolveToSignalObject=off  FilterRTWStateStorageClass=Auto  ParallelPVariant=InternalParameters  IdealPVariant=Disabled  IVariant=InternalParameters  DVariant=Disabled  IntegratorVariant=Discrete  SatVariant=Disabled  AWVariant=Passthrough  PCopyVariant=Disabled  TRVariant=Disabled  FdbkBlocksVariant=Forward  IdealPFdbkVariant=Disabled  SatFdbkVariant=Disabled  DerivativeFilterVariant=Disabled  NVariant=Disabled  NCopyVariant=Disabled_SignalSpec  FilterICVariant=Disabled  IntegratorICVariant=InternalICs  ExternalResetVariant=Disabled  TRSumVariant=Passthrough  SumFdbkVariant=Disabled  SumVariant=Sum_PI  TsampFilterVariant=InternalTs  TsampNgainVariant=Passthrough  TsampIntegralVariant=Disabled_SignalSpec  ExternalSaturationOutDataTypeStr=Inherit: Same as second input  DerivativeSourceVariant=Disabled
  Scope9 : Scope
  Sum16 : Sum  Inputs=|+-
  i(t)3 : Scope
  I(t) : Outport
  wires:
  Sum16/1 -> PID Controller1/1  "e(i)"
  PID Controller1/1 -> Scope9/1, Chart1/4(x)  "U"
  i0(t)/1 -> Sum16/1  "i"
  Chart3/1(y) -> Delay/1, i(t)3/1, I(t)/1
  Constant7/1 -> Chart3/2(T)
  Constant6/1 -> Chart3/1(k)
  Constant5/1 -> Chart3/3(dt)
  Chart1/1(y) -> Chart3/4(x)
  Constant1/1 -> Chart1/1(k)
  Constant2/1 -> Chart1/2(T)
  Constant3/1 -> Chart1/3(dt)
  Delay/1 -> Sum16/2
  Chart1/3(k2) -> Display/1
  Chart1/2(k1) -> Display1/1
  Chart3/3(k2) -> Display2/1
  Chart3/2(k1) -> Display3/1

== system Kurs/Subsystem5 ==
  i0(t) : Inport
  1/(rя*(Ts+1)) : TransferFcn  Numerator=[1/Rya]  Denominator=[Tya 1]
  PID Controller9 : slpidlib/PID Controller  Controller=PI  Form=Parallel  TimeDomain=Continuous-time  UseExternalTs=off  SampleTime=treg  IntegratorMethod=Forward Euler  FilterMethod=Forward Euler  ControllerParametersSource=internal  P=Tya*Rya/(2*Kpr*Tpr)  I=1/Tya  UseKiTs=off  D=-544.981619005016  UseExternalDerivativeSource=off  N=0.000737427491300299  UseFilter=on  TunerSelectOption=Transfer Function Based (PID Tuner App)  InitialConditionSource=internal  InitialConditionForIntegrator=0  InitialConditionForFilter=0  DifferentiatorICPrevScaledInput=0  ExternalReset=none  TrackingMode=off  Kt=1  LimitOutput=off  SatLimitsSource=internal  UpperSaturationLimit=12  LowerSaturationLimit=-12  LinearizeAsGain=on  AntiWindupMode=none  Kb=1  LimitIntegrator=off  UpperIntegratorSaturationLimit=inf  LowerIntegratorSaturationLimit=-inf  POutMin=[]  POutMax=[]  IOutMin=[]  IOutMax=[]  DOutMin=[]  DOutMax=[]  NOutMin=[]  NOutMax=[]  SumOutMin=[]  SumOutMax=[]  SaturationOutMin=[]  SaturationOutMax=[]  PParamMin=[]  PParamMax=[]  IParamMin=[]  IParamMax=[]  DParamMin=[]  DParamMax=[]  NParamMin=[]  NParamMax=[]  KbParamMin=[]  KbParamMax=[]  KtParamMin=[]  KtParamMax=[]  KbOutMin=[]  KbOutMax=[]  KtOutMin=[]  KtOutMax=[]  IntegratorOutMin=[]  IntegratorOutMax=[]  FilterOutMin=[]  FilterOutMax=[]  SumI1OutMin=[]  SumI1OutMax=[]  SumI2OutMin=[]  SumI2OutMax=[]  SumI3OutMin=[]  SumI3OutMax=[]  SumI4OutMin=[]  SumI4OutMax=[]  SumDOutMin=[]  SumDOutMax=[]  DifferentiatorOutMin=[]  DifferentiatorOutMax=[]  FilterDiffOutCoefMin=[]  FilterDiffOutCoefMax=[]  ReciprocalOutMin=[]  ReciprocalOutMax=[]  SumDenOutMin=[]  SumDenOutMax=[]  SumNumOutMin=[]  SumNumOutMax=[]  DivideOutMin=[]  DivideOutMax=[]  UdiffTsProdOutMin=[]  UdiffTsProdOutMax=[]  NTsProdOutMin=[]  NTsProdOutMax=[]  UintegralTsProdOutMin=[]  UintegralTsProdOutMax=[]  UngainTsProdOutMin=[]  UngainTsProdOutMax=[]  ClampingZeroOutDataTypeStr=Inherit: Inherit via back propagation  ClampingZeroOutMin=[]  ClampingZeroOutMax=[]  FilterDenConstantOutDataTypeStr=Inherit: Inherit via back propagation  FilterDenConstantOutMin=[]  FilterDenConstantOutMax=[]  PCopyOutDataTypeStr=Inherit: Inherit via back propagation  PCopyOutMin=[]  PCopyOutMax=[]  NCopyOutDataTypeStr=Inherit: Inherit via back propagation  NCopyOutMin=[]  NCopyOutMax=[]  IntegratorContinuousStateAttributes=''  IntegratorStateMustResolveToSignalObject=off  IntegratorRTWStateStorageClass=Auto  FilterContinuousStateAttributes=''  FilterStateMustResolveToSignalObject=off  FilterRTWStateStorageClass=Auto  ParallelPVariant=InternalParameters  IdealPVariant=Disabled  IVariant=InternalParameters  DVariant=Disabled  IntegratorVariant=Continuous  SatVariant=Disabled  AWVariant=Passthrough  PCopyVariant=Disabled  TRVariant=Disabled  FdbkBlocksVariant=Forward  IdealPFdbkVariant=Disabled  SatFdbkVariant=Disabled  DerivativeFilterVariant=Disabled  NVariant=Disabled  NCopyVariant=Disabled_SignalSpec  FilterICVariant=Disabled  IntegratorICVariant=InternalICs  ExternalResetVariant=Disabled  TRSumVariant=Passthrough  SumFdbkVariant=Disabled  SumVariant=Sum_PI  TsampFilterVariant=InternalTs  TsampNgainVariant=Passthrough  TsampIntegralVariant=Disabled_SignalSpec  ExternalSaturationOutDataTypeStr=Inherit: Same as second input  DerivativeSourceVariant=Disabled
  Scope9 : Scope
  Sum16 : Sum  Inputs=|+-
  i(t)1 : Scope
  i(t)3 : Scope
  kt/(Ts+1) : TransferFcn  Numerator=[Kpr]  Denominator=[Tpr 1]
  I(t) : Outport
  wires:
  Sum16/1 -> PID Controller9/1  "e(i)"
  PID Controller9/1 -> Scope9/1, i(t)1/1, kt/(Ts+1)/1  "U"
  i0(t)/1 -> Sum16/1  "i"
  1/(rя*(Ts+1))/1 -> Sum16/2, i(t)3/1, I(t)/1
  kt/(Ts+1)/1 -> 1/(rя*(Ts+1))/1

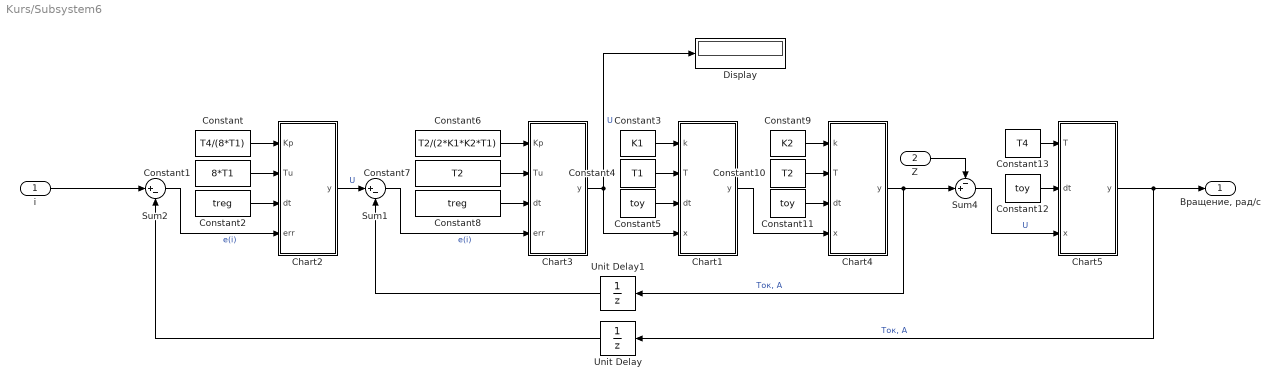
== system Kurs/Subsystem6 ==
  i : Inport
  Z : Inport  Port=2
  Chart1 : Stateflow chart  TreatAsAtomicUnit=on  SystemSampleTime=toy
  Chart2 : Stateflow chart  TreatAsAtomicUnit=on  SystemSampleTime=treg
  Chart3 : Stateflow chart  TreatAsAtomicUnit=on  SystemSampleTime=treg
  Chart4 : Stateflow chart  TreatAsAtomicUnit=on  SystemSampleTime=toy
  Chart5 : Stateflow chart  TreatAsAtomicUnit=on  SystemSampleTime=toy
  Constant : Constant  Value=T4/(8*T1)
  Constant1 : Constant  Value=8*T1
  Constant10 : Constant  Value=T2
  Constant11 : Constant  Value=toy
  Constant12 : Constant  Value=toy
  Constant13 : Constant  Value=T4
  Constant2 : Constant  Value=treg
  Constant3 : Constant  Value=K1
  Constant4 : Constant  Value=T1
  Constant5 : Constant  Value=toy
  Constant6 : Constant  Value=T2/(2*K1*K2*T1)
  Constant7 : Constant  Value=T2
  Constant8 : Constant  Value=treg
  Constant9 : Constant  Value=K2
  Display : Display
  Sum1 : Sum  Inputs=|+-
  Sum2 : Sum  Inputs=|+-
  Sum4 : Sum  Inputs=-+|
  Unit Delay : UnitDelay  SampleTime=-1  HasFrameUpgradeWarning=on
  Unit Delay1 : UnitDelay  SampleTime=-1  HasFrameUpgradeWarning=on
  "Вращение, рад/с" : Outport
  wires:
  Chart4/1(y) -> Unit Delay1/1, Sum4/2  "Ток, А"
  Sum1/1 -> Chart3/4(err)  "e(i)"
  Sum2/1 -> Chart2/4(err)  "e(i)"
  i/1 -> Sum2/1
  Chart2/1(y) -> Sum1/1  "U"
  Sum4/1 -> Chart5/3(x)  "U"
  Z/1 -> Sum4/1
  Constant/1 -> Chart2/1(Kp)
  Constant1/1 -> Chart2/2(Tu)
  Constant2/1 -> Chart2/3(dt)
  Constant6/1 -> Chart3/1(Kp)
  Constant7/1 -> Chart3/2(Tu)
  Constant8/1 -> Chart3/3(dt)
  Chart3/1(y) -> Chart1/4(x), Display/1  "U"
  Constant4/1 -> Chart1/2(T)
  Constant5/1 -> Chart1/3(dt)
  Constant3/1 -> Chart1/1(k)
  Chart1/1(y) -> Chart4/4(x)
  Constant9/1 -> Chart4/1(k)
  Constant10/1 -> Chart4/2(T)
  Constant11/1 -> Chart4/3(dt)
  Chart5/1(y) -> Unit Delay/1, "Вращение, рад/с"/1  "Ток, А"
  Constant12/1 -> Chart5/2(dt)
  Constant13/1 -> Chart5/1(T)
  Unit Delay1/1 -> Sum1/2
  Unit Delay/1 -> Sum2/2

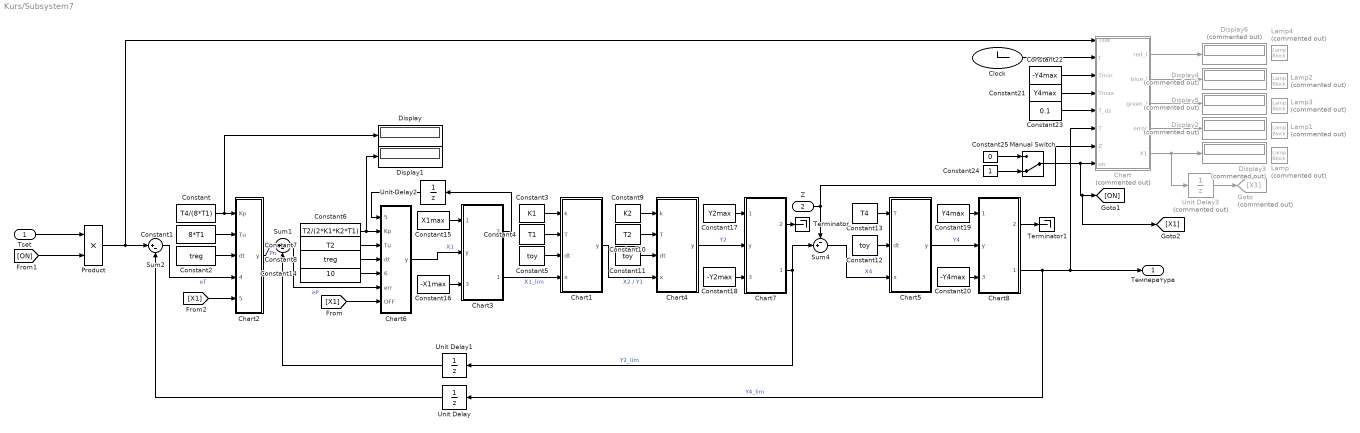
== system Kurs/Subsystem7 ==
  Tset : Inport
  Z : Inport  Port=2
  Chart : Stateflow chart  Commented=on  TreatAsAtomicUnit=on
      settings: PortSchema="{\"entries\":[{\"content\":{\"sides\":[{\"content\":{\"connectorIds\":[\"In8\",\"In1\",\"In2\",\"In3\",\"In5\",\"In4\",\"In6\",\"In7\"]},\"type\":\"ConnectorPlacement.EquallySpacedRectSide\",\"uuid\":\"2a18dcd6-4b0c-4a76-a20c-2dc316dd2b01\"},{\"content\":{\"connectorIds\":[\"Out1\",\"Out2\",\"Out3\",\"Out4\",\"Out5\"],\"side\":\"RIGHT\"},\"type\":\"ConnectorPlacement.EquallySpacedRectSide\",\"uuid\":\"9e7f62ff-8b1d-44fe-8b34-5f319205903d\"},{\"content\":{\"side\":\"TOP\"},\"type\":\"ConnectorPlacement.EquallySpacedRectSide\",\"uuid\":\"488e4df1-10a7-4056-869a-c48ac259fb0e\"}]},\"type\":\"ConnectorPlacement.EquallySpacedConnector\",\"uuid\":\"21634ba7-0beb-4d40-a7b7-ac3b35c407ea\"}],\"packageUris\":[\"http://schema.mathworks.com/mf0/Connector/R2020b\"],\"version\":\"1.0\"}"
  Chart1 : Stateflow chart  TreatAsAtomicUnit=on  SystemSampleTime=toy
  Chart2 : Stateflow chart  TreatAsAtomicUnit=on  SystemSampleTime=treg
  Chart3 : Stateflow chart  TreatAsAtomicUnit=on  SystemSampleTime=treg
      settings: PortSchema="{\"entries\":[{\"content\":{\"sides\":[{\"content\":{\"connectorIds\":[\"In1\",\"In2\",\"In3\"]},\"type\":\"ConnectorPlacement.EquallySpacedRectSide\",\"uuid\":\"06dc2d10-fdc8-420b-b9cd-f5fc9c52f6ec\"},{\"content\":{\"connectorIds\":[\"Out2\",\"Out1\"],\"side\":\"RIGHT\"},\"type\":\"ConnectorPlacement.EquallySpacedRectSide\",\"uuid\":\"6c618a25-ba21-4ff8-999c-a9529d925b85\"},{\"content\":{\"side\":\"TOP\"},\"type\":\"ConnectorPlacement.EquallySpacedRectSide\",\"uuid\":\"fb5392fe-c913-4872-919e-93e45aee3608\"}]},\"type\":\"ConnectorPlacement.EquallySpacedConnector\",\"uuid\":\"af73c6a6-6f26-4653-9043-b34907f5f2e4\"}],\"packageUris\":[\"http://schema.mathworks.com/mf0/Connector/R2020b\"],\"version\":\"1.0\"}"
  Chart4 : Stateflow chart  TreatAsAtomicUnit=on  SystemSampleTime=toy
  Chart5 : Stateflow chart  TreatAsAtomicUnit=on  SystemSampleTime=toy
  Chart6 : Stateflow chart  TreatAsAtomicUnit=on  SystemSampleTime=treg
      settings: PortSchema="{\"entries\":[{\"content\":{\"sides\":[{\"content\":{\"connectorIds\":[\"In5\",\"In1\",\"In2\",\"In3\",\"In6\",\"In4\",\"In7\"]},\"type\":\"ConnectorPlacement.EquallySpacedRectSide\",\"uuid\":\"b164ad06-1259-4e4e-9be1-6467b125c0e4\"},{\"content\":{\"connectorIds\":[\"Out1\"],\"side\":\"RIGHT\"},\"type\":\"ConnectorPlacement.EquallySpacedRectSide\",\"uuid\":\"0593e984-4c4d-48f3-925e-b61cefc7aa48\"},{\"content\":{\"side\":\"TOP\"},\"type\":\"ConnectorPlacement.EquallySpacedRectSide\",\"uuid\":\"e7a407e5-6ce2-46ef-876b-9c67a31d7a68\"}]},\"type\":\"ConnectorPlacement.EquallySpacedConnector\",\"uuid\":\"345a9212-fd2f-406e-95cd-4fdf60a3ef4b\"}],\"packageUris\":[\"http://schema.mathworks.com/mf0/Connector/R2020b\"],\"version\":\"1.0\"}"
  Chart7 : Stateflow chart  TreatAsAtomicUnit=on  SystemSampleTime=toy
      settings: PortSchema="{\"entries\":[{\"content\":{\"sides\":[{\"content\":{\"connectorIds\":[\"In1\",\"In2\",\"In3\"]},\"type\":\"ConnectorPlacement.EquallySpacedRectSide\",\"uuid\":\"06dc2d10-fdc8-420b-b9cd-f5fc9c52f6ec\"},{\"content\":{\"connectorIds\":[\"Out2\",\"Out1\"],\"side\":\"RIGHT\"},\"type\":\"ConnectorPlacement.EquallySpacedRectSide\",\"uuid\":\"6c618a25-ba21-4ff8-999c-a9529d925b85\"},{\"content\":{\"side\":\"TOP\"},\"type\":\"ConnectorPlacement.EquallySpacedRectSide\",\"uuid\":\"fb5392fe-c913-4872-919e-93e45aee3608\"}]},\"type\":\"ConnectorPlacement.EquallySpacedConnector\",\"uuid\":\"af73c6a6-6f26-4653-9043-b34907f5f2e4\"}],\"packageUris\":[\"http://schema.mathworks.com/mf0/Connector/R2020b\"],\"version\":\"1.0\"}"
  Chart8 : Stateflow chart  TreatAsAtomicUnit=on  SystemSampleTime=toy
      settings: PortSchema="{\"entries\":[{\"content\":{\"sides\":[{\"content\":{\"connectorIds\":[\"In1\",\"In2\",\"In3\"]},\"type\":\"ConnectorPlacement.EquallySpacedRectSide\",\"uuid\":\"06dc2d10-fdc8-420b-b9cd-f5fc9c52f6ec\"},{\"content\":{\"connectorIds\":[\"Out2\",\"Out1\"],\"side\":\"RIGHT\"},\"type\":\"ConnectorPlacement.EquallySpacedRectSide\",\"uuid\":\"6c618a25-ba21-4ff8-999c-a9529d925b85\"},{\"content\":{\"side\":\"TOP\"},\"type\":\"ConnectorPlacement.EquallySpacedRectSide\",\"uuid\":\"fb5392fe-c913-4872-919e-93e45aee3608\"}]},\"type\":\"ConnectorPlacement.EquallySpacedConnector\",\"uuid\":\"af73c6a6-6f26-4653-9043-b34907f5f2e4\"}],\"packageUris\":[\"http://schema.mathworks.com/mf0/Connector/R2020b\"],\"version\":\"1.0\"}"
  Clock : Clock
  Constant : Constant  Value=T4/(8*T1)
  Constant1 : Constant  Value=8*T1
  Constant10 : Constant  Value=T2
  Constant11 : Constant  Value=toy
  Constant12 : Constant  Value=toy
  Constant13 : Constant  Value=T4
  Constant14 : Constant  Value=10
  Constant15 : Constant  Value=X1max
  Constant16 : Constant  Value=-X1max
  Constant17 : Constant  Value=Y2max
  Constant18 : Constant  Value=-Y2max
  Constant19 : Constant  Value=Y4max
  Constant2 : Constant  Value=treg
  Constant20 : Constant  Value=-Y4max
  Constant21 : Constant  Value=Y4max
  Constant22 : Constant  Value=-Y4max
  Constant23 : Constant  Value=0.1
  Constant24 : Constant
  Constant25 : Constant  Value=0
  Constant3 : Constant  Value=K1
  Constant4 : Constant  Value=T1
  Constant5 : Constant  Value=toy
  Constant6 : Constant  Value=T2/(2*K1*K2*T1)
  Constant7 : Constant  Value=T2
  Constant8 : Constant  Value=treg
  Constant9 : Constant  Value=K2
  Display : Display
  Display1 : Display
  Display{2..6} (5 alike) : Display  Commented=on
  Goto : Goto  Commented=on  GotoTag=X1
  Lamp : LampBlock  Commented=on  LabelPosition=Hide  Icon=Check1
  Lamp1 : LampBlock  Commented=on  LabelPosition=Hide  Icon=Check1
  Lamp2 : LampBlock  Commented=on  LabelPosition=Hide
  Lamp3 : LampBlock  Commented=on  LabelPosition=Hide
  Lamp4 : LampBlock  Commented=on  LabelPosition=Hide
  Manual Switch : ManualSwitch  CurrentSetting=0
  Product : Product
  Sum1 : Sum  Inputs=|+-
  Sum2 : Sum  Inputs=|+-
  Sum4 : Sum  Inputs=-+|
  Terminator : Terminator
  Terminator1 : Terminator
  Unit Delay : UnitDelay  SampleTime=treg  HasFrameUpgradeWarning=on
  Unit Delay1 : UnitDelay  SampleTime=treg  HasFrameUpgradeWarning=on
  Unit Delay2 : UnitDelay  SampleTime=treg  HasFrameUpgradeWarning=on
  Unit Delay3 : UnitDelay  Commented=on  SampleTime=treg  HasFrameUpgradeWarning=on
  Температура : Outport
  wires:
  Sum1/1 -> Chart6/4(err)  "eP"
  Sum2/1 -> Chart2/4(err)  "eT"
  Tset/1 -> Product/1
  Chart2/1(y) -> Sum1/1  "Pn"
  Sum4/1 -> Chart5/3(x)  "X4"
  Z/1 -> Sum4/1, Chart/6(Z)
  Constant/1 -> Display/1, Chart2/1(Kp)
  Constant1/1 -> Chart2/2(Tu)
  Constant2/1 -> Chart2/3(dt)
  Constant6/1 -> Display1/1, Chart6/1(Kp)
  Constant7/1 -> Chart6/2(Tu)
  Constant8/1 -> Chart6/3(dt)
  Constant4/1 -> Chart1/2(T)
  Constant5/1 -> Chart1/3(dt)
  Constant3/1 -> Chart1/1(k)
  Chart1/1(y) -> Chart4/4(x)  "X2 / Y1"
  Constant9/1 -> Chart4/1(k)
  Constant10/1 -> Chart4/2(T)
  Constant11/1 -> Chart4/3(dt)
  Constant12/1 -> Chart5/2(dt)
  Constant13/1 -> Chart5/1(T)
  Unit Delay/1 -> Sum2/2
  Constant14/1 -> Chart6/6(Kaw)
  Unit Delay2/1 -> Chart6/5(ErrSat)
  Chart7/1(y_lim) -> Unit Delay1/1, Sum4/2  "Y2_lim"
  Chart6/1(y) -> Chart3/2(y)  "X1"
  Chart3/1(y_lim) -> Chart1/4(x)  "X1_lim"
  Constant15/1 -> Chart3/1(Ymax)
  Constant16/1 -> Chart3/3(Ymin)
  Chart4/1(y) -> Chart7/2(y)  "Y2"
  Chart7/2(ErrSat) -> Terminator/1
  Constant17/1 -> Chart7/1(Ymax)
  Constant18/1 -> Chart7/3(Ymin)
  Chart5/1(y) -> Chart8/2(y)  "Y4"
  Chart8/1(y_lim) -> Температура/1, Chart/4(T), Unit Delay/1  "Y4_lim"
  Chart8/2(ErrSat) -> Terminator1/1
  Constant19/1 -> Chart8/1(Ymax)
  Constant20/1 -> Chart8/3(Ymin)
  Chart3/2(ErrSat) -> Unit Delay2/1
  Clock/1 -> Chart/1(t)
  Constant23/1 -> Chart/5(T_dz)
  Chart/4(error) -> Display2/1
  Chart/5(X1) -> Unit Delay3/1, Display3/1
  Chart/3(green_l) -> Display5/1
  Chart/2(blue_l) -> Display4/1
  Chart/1(red_l) -> Display6/1
  Manual Switch/1 -> [X1], [ON], Chart/7(on)
  Constant24/1 -> Manual Switch/2
  Constant25/1 -> Manual Switch/1
  Constant22/1 -> Chart/2(Tmin)
  Constant21/1 -> Chart/3(Tmax)
  Unit Delay1/1 -> Sum1/2
  Product/1 -> Chart/8(Tset), Sum2/1
  [ON] -> Product/2
  [X1] -> Chart2/5(OFF)
  [X1] -> Chart6/7(OFF)
  Unit Delay3/1 -> Goto/1

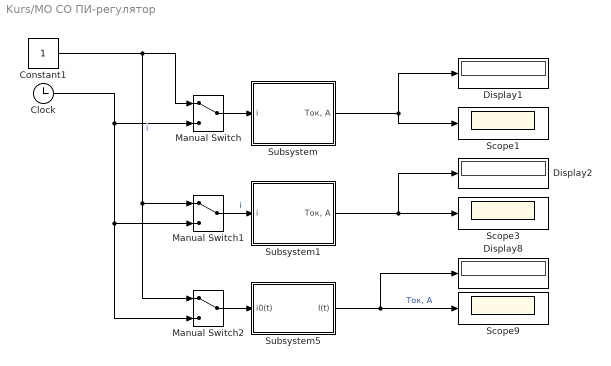
== system Kurs/МО СО ПИ-регулятор ==
  Clock : Clock
  Constant1 : Constant
  Display1 : Display
  Display2 : Display
  Display8 : Display
  Manual Switch : ManualSwitch
  Manual Switch1 : ManualSwitch
  Manual Switch2 : ManualSwitch
  Scope1 : Scope
  Scope3 : Scope
  Scope9 : Scope
  Subsystem : Subsystem
      mask Display: disp('МО контур тока');
  Subsystem1 : Subsystem
      mask Display: disp('СО контур тока');
  Subsystem5 : Subsystem  mask{Kpr=Kpr, Tpr=Tpr, Rya=Rya, Tya=Tya, Cm=c, Ce=c, Kot=Kot, Koc=Koc, treg=0.001, toy=Tpr / 100}
      mask prompts: Kpr "Коэффициент усиления преобразователя"; Tpr "Постоянная времени преобразователя"; Rya "Коэффициент усиления тока (1/Rya)"; Tya "Постоянная времени тока"; Cm "Постоянный конструктивный коэффициент (коэффициент связи)"; Ce "Постоянный конструктивный коэффициент (u = Ce*w)"; Kot "Коэффициент обратной связи тока"; Koc "Коэффициент обратной связи угловой скорости"; treg "Шаг дискретизации регуляторов"; toy "Шаг дискретизации ОУ"
      mask Display: disp('ПИ (дискрет)');
  wires:
  Constant1/1 -> Manual Switch1/1, Manual Switch2/1, Manual Switch/1  "i"
  Subsystem/1("Ток, А") -> Display1/1, Scope1/1
  Subsystem1/1("Ток, А") -> Display2/1, Scope3/1
  Manual Switch1/1 -> Subsystem1/1(i)  "i"
  Manual Switch/1 -> Subsystem/1(i)
  Clock/1 -> Manual Switch2/2, Manual Switch1/2, Manual Switch/2
  Manual Switch2/1 -> Subsystem5/1(i0(t))
  Subsystem5/1(I(t)) -> Display8/1, Scope9/1  "Ток, А"
